simulink model "gm_soc_dvbs2_fpga"  (R2025b)
settings: Solver=FixedStepDiscrete  StartTime=0.0  StopTime=0  RelTol=1e-3
InitFcn:
  | soc_dvbs2_init;
undefined symbols (not defined in the file or in its folder): Add, coefficientsLog, coefficientsSqrt1, coefficientsSqrt2, dataBits, designMultirateFIR, noisePow, Shift, soc_dvbs2_designFIRFilter, soc_dvbs2_txPacketBits, syncWord, txDataOut, txFiltCoeff, XData
libraries: simulink x304, hdlsllib x265, dspsigops x15, dsphdlfiltering2 x8, hdlmdlgenlib x6, dsphdlsigops2 x5, commseqgen3 x5, dsphdlmathfun2 x3, hwlogicconnlib x2, whdledac x2, commhdlcrc x2, whdlutilities x1
(part 1 of 36)
settings Model: DataDictionary=dvbs2hdlReceiverData.sldd  SimulationMode=accelerator  Creator=The MathWorks, Inc.  LastModifiedBy=AEDemo
settings SolverCC: PositivePriorityOrder=on  MaxZcPerStep=1.0
settings DataIOCC: ReturnWorkspaceOutputs=off
settings OptimizationCC: BlockReduction=off  ConditionallyExecuteInputs=off  DefaultParameterBehavior=Inlined  InheritOutputTypeSmallerThanSingle=on  EnhancedBackFolding=on  PassReuseOutputArgsAs=Individual arguments  ZeroExternalMemoryAtStartup=off  ZeroInternalMemoryAtStartup=off  MaxStackSize=64  OptimizeBlockOrder=speed  DifferentSizesBufferReuse=on  OptimizationCustomize=off  EfficientTunableParamExpr=on
settings DebuggingCC: ArtificialAlgebraicLoopMsg=error  InheritedTsInSrcMsg=none  SingleTaskRateTransMsg=error  ParameterTunabilityLossMsg=error  UnconnectedInputMsg=warning  UnconnectedOutputMsg=warning  UnconnectedLineMsg=warning  SubsystemReferenceDiagnosticForUnitTest=warning
settings HardwareCC: ProdBitPerPointer=32.0  ProdBitPerSizeT=32.0  ProdBitPerPtrDiffT=32.0  ProdLargestAtomicFloat=None  ProdIntDivRoundTo=Undefined  ProdEndianess=Unspecified  ProdWordSize=32.0  ProdHWDeviceType=ASIC/FPGA->ASIC/FPGA  TargetBitPerPointer=64.0  TargetBitPerSizeT=64.0  TargetBitPerPtrDiffT=64.0  TargetLongLongMode=on  TargetIntDivRoundTo=Zero  TargetEndianess=LittleEndian  TargetWordSize=64.0  TargetHWDeviceType=Custom Processor->MATLAB Host Computer  ProdEqTarget=off  HardwareBoardFeatureSet=SoCBlockset
settings ModelReferenceCC: EnableRefExpFcnMdlSchedulingChecks=on
settings RTWCC: SystemTargetFile=ert.tlc  HardwareBoard=Xilinx Zynq UltraScale+ RFSoC ZCU111 Evaluation Kit  TLCOptions="-aInlineSetEventsForThisBaseRateFcn=TLC_FALSE -aSuppressMultiTaskScheduler=TLC_FALSE  -aRateBasedStepFcn=0"  TemplateMakefile=ert_default_tmf  Toolchain=Linaro AArch64 Linux v6.3.1  GPUComputeCapability=3.5  DLArmComputeVersion=19.05  Description=Embedded Coder
settings CodeAppCC: ForceParamTrailComments=on  IgnoreCustomStorageClasses=off  OperatorAnnotations=on  SimulinkDataObjDesc=on  SFDataObjDesc=on  InsertBlockDesc=on

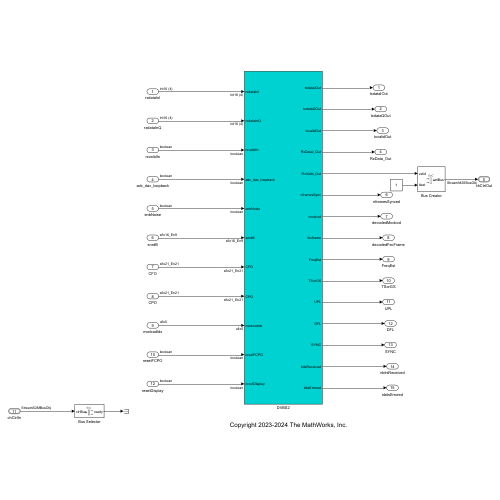
[thumbnail: Simulink's stored preview of the top-level diagram]
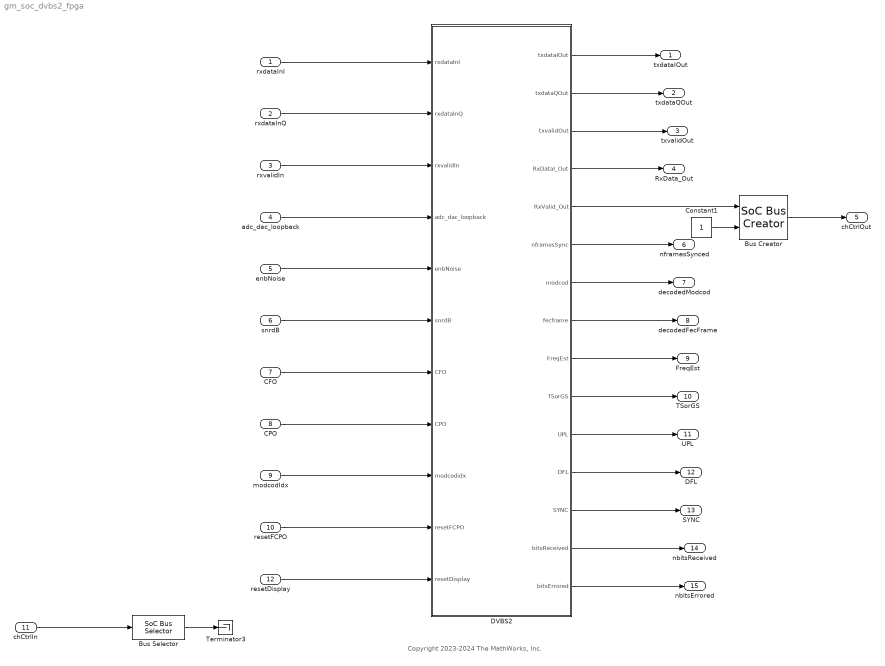
== system gm_soc_dvbs2_fpga ==
  note: Copyright 2023-2024 The MathWorks, Inc.
  rxdataInI : Inport  OutDataTypeStr=int16  PortDimensions=4  LockScale=on
  rxdataInQ : Inport  Port=2  OutDataTypeStr=int16  PortDimensions=4  LockScale=on
  rxvalidIn : Inport  Port=3  OutDataTypeStr=boolean  LockScale=on
  adc_dac_loopback : Inport  Port=4  OutDataTypeStr=boolean  LockScale=on
  enbNoise : Inport  Port=5  OutDataTypeStr=boolean
  snrdB : Inport  Port=6  OutDataTypeStr=fixdt(1,16,9)
  CFO : Inport  Port=7  OutDataTypeStr=fixdt(1,21,21)
  CPO : Inport  Port=8  OutDataTypeStr=fixdt(1,21,21)
  modcodIdx : Inport  Port=9  OutDataTypeStr=fixdt(0,5,0)
  resetFCPO : Inport  Port=10  OutDataTypeStr=boolean
  chCtrlIn : Inport  Port=11  OutDataTypeStr=Bus: StreamS2MBusObj  BusOutputAsStruct=on
  resetDisplay : Inport  Port=12  OutDataTypeStr=boolean
  Bus Creator : hwlogicconnlib/SoC Bus Creator  Protocol=Data stream  ctrltype=Valid
  Bus Selector : hwlogicconnlib/SoC Bus Selector  Protocol=Data stream  ctrltype=Ready
  Constant1 : Constant  OutDataTypeStr=boolean  SampleTime=-1
  DVBS2 : Subsystem
      mask init:
      | coe = reshape(double([0;-4.6183113992051936e-06;-1.117761640887225e-05;-1.8610264502005432e-05;-2.5134586135631012e-05;-2.8494281690666197e-05;-2.6396828793275159e-05;-1.7094212558802163e-05;0;2.3798193576966866e-05;5.1281160242202183e-05;7.7621978262434297e-05;9.6759426664120416e-05;0.00010240229300393402;8.9344614218077133e-05;5.4875700118949183e-05;0;-6.9839082210680138e-05;-0.00014479661323607565;-0.00021158452917708308;-0.00025535069106550544;-0.00026228714374322104;-0.00022258805927027799;-0.00013323230495695704;0;0.00016182578767055206;0.00032846175385096581;0.00047045611576184863;0.00055713851457530922;0.00056212565121518737;0.00046901918553962478;0.00027624866838952986;0;-0.00032564179486838622;-0.00065182310286710399;-0.00092127787309319298;-0.0010772534348943575;-0.0010737727700273478;-0.00088556645390392634;-0.00051581896090765534;0;0.00059548767193795277;0.0011803558710661007;0.0016527320270369871;0.0019152679330965558;0.0018927324805381538;0.0015481870327877928;0.00089470695834941306;0;-0.0010178225878206132;-0.0020037400552054292;-0.0027874356824117317;-0.003210329988021943;-0.0031540624117984395;-0.0025657163651900345;-0.0014750752642111449;0;0.0016624165446378462;0.0032591192839069179;0.004516568581586773;0.0051838984346123896;0.0050774264697459942;0.0041192521414141594;0.00236285754179665;0;-0.0026543507866759182;-0.0051990251084333425;-0.0072020238234656924;-0.0082672928192007358;-0.008103373957295627;-0.006583111539570221;-0.0037839040415292386;0;0.0042781252851152524;0.0084176358598320178;0.011725660574630552;0.013550476647788677;0.013388189369997498;0.010979501242341257;0.006381274941685413;0;-0.007421229604153888;-0.01486456304340213;-0.021143584622178104;-0.02504275058758609;-0.025473530942547201;-0.021627310017882196;-0.013104323383225537;0;0.017065133989980476;0.036978919264451952;0.05823318062093958;0.079072012081405949;0.097675998716952317;0.11236045936950929;0.12176343577287731;0.125;0.12176343577287731;0.11236045936950929;0.097675998716952317;0.079072012081405949;0.05823318062093958;0.036978919264451952;0.017065133989980476;0;-0.013104323383225537;-0.021627310017882196;-0.025473530942547201;-0.02504275058758609;-0.021143584622178104;-0.01486456304340213;-0.007421229604153888;0;0.006381274941685413;0.010979501242341257;0.013388189369997498;0.013550476647788677;0.011725660574630552;0.0084176358598320178;0.0042781252851152524;0;-0.0037839040415292386;-0.006583111539570221;-0.008103373957295627;-0.0082672928192007358;-0.0072020238234656924;-0.0051990251084333425;-0.0026543507866759182;0;0.00236285754179665;0.0041192521414141594;0.0050774264697459942;0.0051838984346123896;0.004516568581586773;0.0032591192839069179;0.0016624165446378462;0;-0.0014750752642111449;-0.0025657163651900345;-0.0031540624117984395;-0.003210329988021943;-0.0027874356824117317;-0.0020037400552054292;-0.0010178225878206132;0;0.00089470695834941306;0.0015481870327877928;0.0018927324805381538;0.0019152679330965558;0.0016527320270369871;0.0011803558710661007;0.00059548767193795277;0;-0.00051581896090765534;-0.00088556645390392634;-0.0010737727700273478;-0.0010772534348943575;-0.00092127787309319298;-0.00065182310286710399;-0.00032564179486838622;0;0.00027624866838952986;0.00046901918553962478;0.00056212565121518737;0.00055713851457530922;0.00047045611576184863;0.00032846175385096581;0.00016182578767055206;0;-0.00013323230495695704;-0.00022258805927027799;-0.00026228714374322104;-0.00025535069106550544;-0.00021158452917708308;-0.00014479661323607565;-6.9839082210680138e-05;0;5.4875700118949183e-05;8.9344614218077133e-05;0.00010240229300393402;9.6759426664120416e-05;7.7621978262434297e-05;5.1281160242202183e-05;2.3798193576966866e-05;0;-1.7094212558802163e-05;-2.6396828793275159e-05;-2.8494281690666197e-05;-2.5134586135631012e-05;-1.8610264502005432e-05;-1.117761640887225e-05;-4.6183113992051936e-06]), [1  192]);
      | interp_coeff = reshape(double([0;-2.5762581491757149e-05;-5.8831821680514759e-05;-9.3312161185059878e-05;-0.00012086163085409433;-0.00013205270976779482;-0.00011834743116057382;-7.4366825754989437e-05;0;9.8160915307191784e-05;0.00020653032645552219;0.00030569884691874328;0.00037312606030348193;0.00038710567399410266;0.00033143343994865174;0.00019995023815725909;0;-0.00024611644953130535;-0.00050237406876756942;-0.00072320914773199184;-0.00086038268936497941;-0.00087166788797456607;-0.00073000105198961778;-0.00043141174353976327;0;0.00051149159396842369;0.0010263594832950844;0.0014538625812232689;0.0017033853517477954;0.0017008871462745852;0.0014049583413437243;0.00081947197501865956;0;-0.00094810607847870226;-0.0018808492888220838;-0.0026352624613329868;-0.0030553081816828832;-0.0030202428411423995;-0.0024707286522091098;-0.0014277474612946694;0;0.0016230413454147042;0.0031930796109812462;0.0044380259174111297;0.0051056581078908472;0.0050093785155702775;0.0040683784677133959;0.0023345651421505286;0;-0.0026187539064786284;-0.0051193984472911441;-0.0070718134335119327;-0.0080873994108355395;-0.0078893031903380026;-0.0063716582505391091;-0.0036365506713397764;0;0.0040374115839547997;0.0078540829737719763;0.010798012443441477;0.012292073245047443;0.011937778189025024;0.0095999760380976757;0.0054563636732276643;0;-0.0060102816730613498;-0.011648449375858055;-0.015957241826634484;-0.018102591848754991;-0.017522692405904365;-0.014046537497763033;-0.007959475987989087;0;0.008718104923122711;0.01685235137753412;0.023029139138304663;0.026064622673058715;0.025174843574555367;0.020139852028642682;0.011390947438140097;0;-0.012436079757686049;-0.024006222786136334;-0.032765654100451284;-0.03704666586468406;-0.035752212682362922;-0.028583560689952235;-0.01615969653056519;0;0.017638825193237648;0.034058051458235795;0.046508756928501517;0.052626172604575812;0.050841305470613003;0.040702766275549772;0.023050307008179838;0;-0.025272869236065459;-0.048936761752801212;-0.067046073615192756;-0.07615058129553684;-0.073883911648887329;-0.05943876854292833;-0.033846317708509245;0;0.037602423644390599;0.073384893960547079;0.10143269424548541;0.11635564505557951;0.11415986456169339;0.093003185804921784;0.053716748922668422;0;-0.061764245016254132;-0.12307869991479406;-0.17423577931097833;-0.20545948334743191;-0.20814945771861357;-0.17607037667070338;-0.10632880802090262;0;0.13769341192513965;0.29769467708537439;0.46790031420225453;0.63434243500199439;0.78263423378671237;0.89951021019816191;0.97427716367867034;1;0.97427716367867034;0.89951021019816191;0.78263423378671237;0.63434243500199439;0.46790031420225453;0.29769467708537439;0.13769341192513965;0;-0.10632880802090262;-0.17607037667070338;-0.20814945771861357;-0.20545948334743191;-0.17423577931097833;-0.12307869991479406;-0.061764245016254132;0;0.053716748922668422;0.093003185804921784;0.11415986456169339;0.11635564505557951;0.10143269424548541;0.073384893960547079;0.037602423644390599;0;-0.033846317708509245;-0.05943876854292833;-0.073883911648887329;-0.07615058129553684;-0.067046073615192756;-0.048936761752801212;-0.025272869236065459;0;0.023050307008179838;0.040702766275549772;0.050841305470613003;0.052626172604575812;0.046508756928501517;0.034058051458235795;0.017638825193237648;0;-0.01615969653056519;-0.028583560689952235;-0.035752212682362922;-0.03704666586468406;-0.032765654100451284;-0.024006222786136334;-0.012436079757686049;0;0.011390947438140097;0.020139852028642682;0.025174843574555367;0.026064622673058715;0.023029139138304663;0.01685235137753412;0.008718104923122711;0;-0.007959475987989087;-0.014046537497763033;-0.017522692405904365;-0.018102591848754991;-0.015957241826634484;-0.011648449375858055;-0.0060102816730613498;0;0.0054563636732276643;0.0095999760380976757;0.011937778189025024;0.012292073245047443;0.010798012443441477;0.0078540829737719763;0.0040374115839547997;0;-0.0036365506713397764;-0.0063716582505391091;-0.0078893031903380026;-0.0080873994108355395;-0.0070718134335119327;-0.0051193984472911441;-0.0026187539064786284;0;0.0023345651421505286;0.0040683784677133959;0.0050093785155702775;0.0051056581078908472;0.0044380259174111297;0.0031930796109812462;0.0016230413454147042;0;-0.0014277474612946694;-0.0024707286522091098;-0.0030202428411423995;-0.0030553081816828832;-0.0026352624613329868;-0.0018808492888220838;-0.00094810607847870226;0;0.00081947197501865956;0.0014049583413437243;0.0017008871462745852;0.0017033853517477954;0.0014538625812232689;0.0010263594832950844;0.00051149159396842369;0;-0.00043141174353976327;-0.00073000105198961778;-0.00087166788797456607;-0.00086038268936497941;-0.00072320914773199184;-0.00050237406876756942;-0.00024611644953130535;0;0.00019995023815725909;0.00033143343994865174;0.00038710567399410266;0.00037312606030348193;0.00030569884691874328;0.00020653032645552219;9.8160915307191784e-05;0;-7.4366825754989437e-05;-0.00011834743116057382;-0.00013205270976779482;-0.00012086163085409433;-9.3312161185059878e-05;-5.8831821680514759e-05;-2.5762581491757149e-05]), [1  256]);
  Terminator3 : Terminator
  txdataIOut : Outport
  txdataQOut : Outport  Port=2
  txvalidOut : Outport  Port=3
  RxData_Out : Outport  Port=4
  chCtrlOut : Outport  Port=5  OutDataTypeStr=Bus: StreamM2SBusObj  VectorParamsAs1DForOutWhenUnconnected=off  BusOutputAsStruct=on
  nframesSynced : Outport  Port=6
  decodedModcod : Outport  Port=7
  decodedFecFrame : Outport  Port=8
  FreqEst : Outport  Port=9
  TSorGS : Outport  Port=10
  UPL : Outport  Port=11
  DFL : Outport  Port=12
  SYNC : Outport  Port=13
  nbitsReceived : Outport  Port=14
  nbitsErrored : Outport  Port=15
  wires:
  resetDisplay/1 -> DVBS2/11(resetDisplay)
  DVBS2/15(bitsErrored) -> nbitsErrored/1
  DVBS2/14(bitsReceived) -> nbitsReceived/1
  DVBS2/12(DFL) -> DFL/1
  DVBS2/10(TSorGS) -> TSorGS/1
  DVBS2/13(SYNC) -> SYNC/1
  DVBS2/11(UPL) -> UPL/1
  DVBS2/2(txdataQOut) -> txdataQOut/1
  DVBS2/1(txdataIOut) -> txdataIOut/1
  CFO/1 -> DVBS2/7(CFO)
  Bus Selector/1 -> Terminator3/1
  chCtrlIn/1 -> Bus Selector/1
  Constant1/1 -> Bus Creator/2
  DVBS2/5(RxValid_Out) -> Bus Creator/1
  Bus Creator/1 -> chCtrlOut/1
  DVBS2/4(RxDataI_Out) -> RxData_Out/1
  resetFCPO/1 -> DVBS2/10(resetFCPO)
  DVBS2/9(FreqEst) -> FreqEst/1
  DVBS2/8(fecframe) -> decodedFecFrame/1
  DVBS2/7(modcod) -> decodedModcod/1
  DVBS2/6(nframesSync) -> nframesSynced/1
  DVBS2/3(txvalidOut) -> txvalidOut/1
  enbNoise/1 -> DVBS2/5(enbNoise)
  modcodIdx/1 -> DVBS2/9(modcodidx)
  CPO/1 -> DVBS2/8(CPO)
  snrdB/1 -> DVBS2/6(snrdB)
  adc_dac_loopback/1 -> DVBS2/4(adc_dac_loopback)
  rxvalidIn/1 -> DVBS2/3(rxvalidIn)
  rxdataInQ/1 -> DVBS2/2(rxdataInQ)
  rxdataInI/1 -> DVBS2/1(rxdataInI)

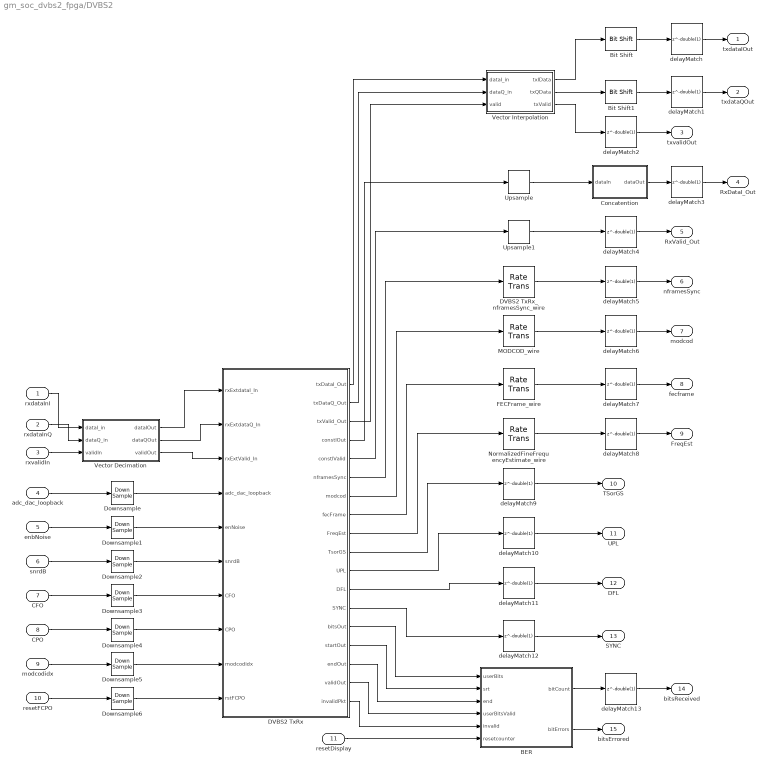
== system gm_soc_dvbs2_fpga/DVBS2 ==
  rxdataInI : Inport  OutDataTypeStr=int16  PortDimensions=[4]  SampleTime=7.8125e-09
  rxdataInQ : Inport  Port=2  OutDataTypeStr=int16  PortDimensions=[4]  SampleTime=7.8125e-09
  rxvalidIn : Inport  Port=3  OutDataTypeStr=boolean  PortDimensions=1  SampleTime=7.8125e-09
  adc_dac_loopback : Inport  Port=4  OutDataTypeStr=boolean  PortDimensions=1  SampleTime=7.8125e-09
  enbNoise : Inport  Port=5  OutDataTypeStr=boolean  PortDimensions=1  SampleTime=7.8125e-09
  snrdB : Inport  Port=6  OutDataTypeStr=fixdt(1, 16, 9)  PortDimensions=1  SampleTime=7.8125e-09
  CFO : Inport  Port=7  OutDataTypeStr=fixdt(1, 21, 21)  PortDimensions=1  SampleTime=7.8125e-09
  CPO : Inport  Port=8  OutDataTypeStr=fixdt(1, 21, 21)  PortDimensions=1  SampleTime=7.8125e-09
  modcodidx : Inport  Port=9  OutDataTypeStr=fixdt(0, 5, 0)  PortDimensions=1  SampleTime=7.8125e-09
  resetFCPO : Inport  Port=10  OutDataTypeStr=boolean  PortDimensions=1  SampleTime=7.8125e-09
  resetDisplay : Inport  Port=11  OutDataTypeStr=boolean  PortDimensions=1  SampleTime=7.8125e-09
  BER : Subsystem
  Bit Shift : hdlsllib/Logic and Bit Operations/Bit Shift  mode=Shift Left Logical  N=double(2)
  Bit Shift1 : hdlsllib/Logic and Bit Operations/Bit Shift  mode=Shift Left Logical  N=double(2)
  Concatention : Subsystem
  DVBS2 TxRx : Subsystem
  DVBS2 TxRx_nframesSync_wire : RateTransition  Integrity=off  Deterministic=off  OutPortSampleTimeOpt=Multiple of input port sample time  OutPortSampleTimeMultiple=1/32
  Downsample{,1..6} (7 alike) : DownSample  N=double(8)  phase=double(0)  RateOptions=Allow multirate processing  AllowArbitraryFixedInput=on
  FECFrame_wire : RateTransition  Integrity=off  Deterministic=off  OutPortSampleTimeOpt=Multiple of input port sample time  OutPortSampleTimeMultiple=1/32
  MODCOD_wire : RateTransition  Integrity=off  Deterministic=off  OutPortSampleTimeOpt=Multiple of input port sample time  OutPortSampleTimeMultiple=1/32
  NormalizedFineFrequencyEstimate_wire : RateTransition  Integrity=off  Deterministic=off  OutPortSampleTimeOpt=Multiple of input port sample time  OutPortSampleTimeMultiple=1/32
  Upsample : dspsigops/Upsample  FactorSource=Dialog parameter  N=double(32)  Nmax=16  phase=double(0)  RateOptions=Allow multirate processing  ic=0  mode=Unused parameter value
  Upsample1 : dspsigops/Upsample  FactorSource=Dialog parameter  N=double(32)  Nmax=16  phase=double(0)  RateOptions=Allow multirate processing  ic=0  mode=Unused parameter value
  Vector Decimation : Subsystem
  Vector Interpolation : Subsystem
  delayMatch{,1..13} (14 alike) : Delay  DelayLength=double(1)  InitialCondition=0  SampleTime=7.8125e-09
  txdataIOut : Outport  SampleTime=7.8125e-09
  txdataQOut : Outport  Port=2  SampleTime=7.8125e-09
  txvalidOut : Outport  Port=3  SampleTime=7.8125e-09
  RxDataI_Out : Outport  Port=4  SampleTime=7.8125e-09
  RxValid_Out : Outport  Port=5  SampleTime=7.8125e-09
  nframesSync : Outport  Port=6  SampleTime=7.8125e-09
  modcod : Outport  Port=7  SampleTime=7.8125e-09
  fecframe : Outport  Port=8  SampleTime=7.8125e-09
  FreqEst : Outport  Port=9  SampleTime=7.8125e-09
  TSorGS : Outport  Port=10  SampleTime=7.8125e-09
  UPL : Outport  Port=11  SampleTime=7.8125e-09
  DFL : Outport  Port=12  SampleTime=7.8125e-09
  SYNC : Outport  Port=13  SampleTime=7.8125e-09
  bitsReceived : Outport  Port=14  SampleTime=7.8125e-09
  bitsErrored : Outport  Port=15  SampleTime=7.8125e-09
  wires:
  Downsample5/1 -> DVBS2 TxRx/9(modcodidx)
  enbNoise/1 -> Downsample1/1
  DVBS2 TxRx_nframesSync_wire/1 -> delayMatch5/1
  rxdataInI/1 -> Vector Decimation/1(dataI_in)
  DVBS2 TxRx/7(modcod) -> MODCOD_wire/1
  CPO/1 -> Downsample4/1
  CFO/1 -> Downsample3/1
  DVBS2 TxRx/2(txDataQ_Out) -> Vector Interpolation/2(dataQ_in)
  Upsample1/1 -> delayMatch4/1
  DVBS2 TxRx/5(constlValid) -> Upsample1/1
  snrdB/1 -> Downsample2/1
  DVBS2 TxRx/3(txValid_Out) -> Vector Interpolation/3(valid)
  adc_dac_loopback/1 -> Downsample/1
  NormalizedFineFrequencyEstimate_wire/1 -> delayMatch8/1
  resetDisplay/1 -> BER/6(resetcounter)
  DVBS2 TxRx/6(nframesSync) -> DVBS2 TxRx_nframesSync_wire/1
  rxvalidIn/1 -> Vector Decimation/3(validIn)
  Bit Shift1/1 -> delayMatch1/1
  DVBS2 TxRx/1(txDataI_Out) -> Vector Interpolation/1(dataI_in)
  resetFCPO/1 -> Downsample6/1
  rxdataInQ/1 -> Vector Decimation/2(dataQ_in)
  DVBS2 TxRx/4(constlOut) -> Upsample/1
  modcodidx/1 -> Downsample5/1
  Vector Decimation/1(dataIOut) -> DVBS2 TxRx/1(rxExtdataI_In)
  Vector Decimation/2(dataQOut) -> DVBS2 TxRx/2(rxExtdataQ_In)
  MODCOD_wire/1 -> delayMatch6/1
  Vector Decimation/3(validOut) -> DVBS2 TxRx/3(rxExtValid_In)
  FECFrame_wire/1 -> delayMatch7/1
  Downsample/1 -> DVBS2 TxRx/4(adc_dac_loopback)
  Downsample1/1 -> DVBS2 TxRx/5(enNoise)
  Downsample2/1 -> DVBS2 TxRx/6(snrdB)
  Downsample4/1 -> DVBS2 TxRx/8(CPO)
  Downsample3/1 -> DVBS2 TxRx/7(CFO)
  Downsample6/1 -> DVBS2 TxRx/10(rstFCPO)
  DVBS2 TxRx/8(fecFrame) -> FECFrame_wire/1
  delayMatch11/1 -> DFL/1
  DVBS2 TxRx/17(validOut) -> BER/4(userBitsValid)
  DVBS2 TxRx/9(FreqEst) -> NormalizedFineFrequencyEstimate_wire/1
  DVBS2 TxRx/10(TsorGS) -> delayMatch9/1
  delayMatch9/1 -> TSorGS/1
  DVBS2 TxRx/18(invalidPkt) -> BER/5(invalid)
  delayMatch7/1 -> fecframe/1
  DVBS2 TxRx/11(UPL) -> delayMatch10/1
  delayMatch5/1 -> nframesSync/1
  DVBS2 TxRx/12(DFL) -> delayMatch11/1
  DVBS2 TxRx/13(SYNC) -> delayMatch12/1
  DVBS2 TxRx/14(bitsOut) -> BER/1(userBits)
  DVBS2 TxRx/15(startOut) -> BER/2(srt)
  Vector Interpolation/2(txQData) -> Bit Shift1/1
  delayMatch13/1 -> bitsReceived/1
  DVBS2 TxRx/16(endOut) -> BER/3(end)
  delayMatch6/1 -> modcod/1
  Vector Interpolation/1(txIData) -> Bit Shift/1
  Vector Interpolation/3(txValid) -> delayMatch2/1
  Upsample/1 -> Concatention/1(dataIn)
  delayMatch10/1 -> UPL/1
  delayMatch12/1 -> SYNC/1
  BER/1(bitCount) -> delayMatch13/1
  BER/2(bitErrors) -> bitsErrored/1
  Bit Shift/1 -> delayMatch/1
  delayMatch2/1 -> txvalidOut/1
  Concatention/1(dataOut) -> delayMatch3/1
  delayMatch4/1 -> RxValid_Out/1
  delayMatch8/1 -> FreqEst/1
  delayMatch/1 -> txdataIOut/1
  delayMatch1/1 -> txdataQOut/1
  delayMatch3/1 -> RxDataI_Out/1

== system gm_soc_dvbs2_fpga/DVBS2/BER ==
  userBits : Inport  OutDataTypeStr=boolean  PortDimensions=1  SampleTime=7.8125e-09
  srt : Inport  Port=2  OutDataTypeStr=boolean  PortDimensions=1  SampleTime=7.8125e-09
  end : Inport  Port=3  OutDataTypeStr=boolean  PortDimensions=1  SampleTime=7.8125e-09
  userBitsValid : Inport  Port=4  OutDataTypeStr=boolean  PortDimensions=1  SampleTime=7.8125e-09
  invalid : Inport  Port=5  OutDataTypeStr=boolean  PortDimensions=1  SampleTime=7.8125e-09
  resetcounter : Inport  Port=6  OutDataTypeStr=boolean  PortDimensions=1  SampleTime=7.8125e-09
  Compare To Constant : simulink/Logic and Bit Operations/Compare To Constant  relop===  const="fi(0,0,32,0,\"hex\",\"00000000\")"  OutDataTypeStr=boolean
  Data Type Conversion1 : DataTypeConversion  OutDataTypeStr=boolean  SampleTime=7.8125e-09  SaturateOnIntegerOverflow=off  RndMeth=Floor
  Delay : Delay  DelayLength=double(1)  InitialCondition=0  SampleTime=7.8125e-09
  Delay1 : Delay  DelayLength=double(1)  InitialCondition=0  SampleTime=7.8125e-09
  Delay4 : Delay  DelayLength=double(1550)  InitialCondition=0  SampleTime=7.8125e-09
  Delay5 : Delay  DelayLength=double(1550)  InitialCondition=0  SampleTime=7.8125e-09
  Delay6 : Delay  DelayLength=double(1550)  InitialCondition=0  SampleTime=7.8125e-09
  HDL Counter : hdlsllib/Sources/HDL Counter  CountType=Free running  CountInit=0  CountStep=1  CountMax=25  CountFromType=Initial value  CountFrom=0  CountResetPort=on  CountLoadPort=off  CountEnbPort=on  CountDirPort=off  CountHitOutputPort=off  CountDataType=Unsigned  CountWordLen=32  CountFracLen=0  CountSampTime=1
  HDL Counter1 : hdlsllib/Sources/HDL Counter  CountType=Free running  CountInit=0  CountStep=1  CountMax=25  CountFromType=Initial value  CountFrom=0  CountResetPort=on  CountLoadPort=off  CountEnbPort=on  CountDirPort=off  CountHitOutputPort=off  CountDataType=Unsigned  CountWordLen=32  CountFracLen=0  CountSampTime=1
  Logical Operator : Logic  AllPortsSameDT=off  OutDataTypeStr=boolean  SampleTime=7.8125e-09
  Logical Operator1 : Logic  Operator=OR  AllPortsSameDT=off  OutDataTypeStr=boolean  SampleTime=7.8125e-09
  Logical Operator2 : Logic  Operator=NOT  Inputs=1  AllPortsSameDT=off  OutDataTypeStr=boolean  SampleTime=7.8125e-09
  Logical Operator3 : Logic  AllPortsSameDT=off  OutDataTypeStr=boolean  SampleTime=7.8125e-09
  Relational Operator : RelationalOperator  Operator=~=  OutDataTypeStr=boolean  SampleTime=7.8125e-09  InputSameDT=off
  Send Payload Data : Subsystem
  Unit Delay Enabled Synchronous : hdlsllib/Discrete/Unit Delay Enabled Synchronous  InitialCondition=double(0)  SampleTime=-1
  Unit Delay Enabled Synchronous1 : hdlsllib/Discrete/Unit Delay Enabled Synchronous  InitialCondition=double(0)  SampleTime=-1
  delayMatch : Delay  DelayLength=double(1)  InitialCondition=0  SampleTime=7.8125e-09
  delayMatch1 : Delay  DelayLength=double(1)  InitialCondition=0  SampleTime=7.8125e-09
  delayMatch2 : Delay  DelayLength=double(1)  InitialCondition=0  SampleTime=7.8125e-09
  bitCount : Outport  SampleTime=7.8125e-09  VectorParamsAs1DForOutWhenUnconnected=off
  bitErrors : Outport  Port=2  SampleTime=7.8125e-09  VectorParamsAs1DForOutWhenUnconnected=off
  wires:
  userBitsValid/1 -> Delay4/1
  Data Type Conversion1/1 -> Relational Operator/2
  invalid/1 -> Unit Delay Enabled Synchronous/1
  srt/1 -> Delay6/1
  end/1 -> Unit Delay Enabled Synchronous/2
  Unit Delay Enabled Synchronous/1 -> Logical Operator2/1
  Logical Operator/1 -> HDL Counter/2
  delayMatch2/1 -> HDL Counter/1
  Logical Operator2/1 -> Unit Delay Enabled Synchronous1/1
  Delay4/1 -> Delay1/1
  Delay6/1 -> Send Payload Data/1(rst), Unit Delay Enabled Synchronous1/2
  Unit Delay Enabled Synchronous1/1 -> Logical Operator3/1
  Delay1/1 -> Logical Operator3/2
  userBits/1 -> Delay5/1
  resetcounter/1 -> Logical Operator1/2, HDL Counter1/1
  Logical Operator3/1 -> delayMatch1/1, HDL Counter1/2, Send Payload Data/2(nxtBit)
  Delay5/1 -> Delay/1
  HDL Counter1/1 -> Compare To Constant/1, bitCount/1
  Delay/1 -> delayMatch/1
  Send Payload Data/1(dataIn) -> Data Type Conversion1/1
  Compare To Constant/1 -> Logical Operator1/1
  delayMatch/1 -> Relational Operator/1
  Logical Operator1/1 -> delayMatch2/1
  delayMatch1/1 -> Logical Operator/1
  Relational Operator/1 -> Logical Operator/2
  HDL Counter/1 -> bitErrors/1

== system gm_soc_dvbs2_fpga/DVBS2/Concatention ==
  dataIn : Inport  OutDataTypeStr=fixdt(1, 18, 14)  PortDimensions=1  SampleTime=7.8125e-09
      settings: SignalType=complex
  Bit Concat : hdlsllib/Logic and Bit Operations/Bit Concat  numInputs=2
  Complex to Real-Imag1 : ComplexToRealImag
  Data Type Conversion : DataTypeConversion  OutDataTypeStr=fixdt(1,16,12)  SaturateOnIntegerOverflow=off  RndMeth=Floor
  Data Type Conversion1 : DataTypeConversion  OutDataTypeStr=int16  ConvertRealWorld=Stored Integer (SI)  SaturateOnIntegerOverflow=off  RndMeth=Floor
  dataOut : Outport  SampleTime=7.8125e-09
  wires:
  dataIn/1 -> Data Type Conversion/1
  Bit Concat/1 -> dataOut/1
  Complex to Real-Imag1/2 -> Bit Concat/2
  Complex to Real-Imag1/1 -> Bit Concat/1
  Data Type Conversion1/1 -> Complex to Real-Imag1/1
  Data Type Conversion/1 -> Data Type Conversion1/1

== system gm_soc_dvbs2_fpga/DVBS2/DVBS2 TxRx ==
  rxExtdataI_In : Inport  OutDataTypeStr=int16  PortDimensions=1  SampleTime=7.8125e-09
  rxExtdataQ_In : Inport  Port=2  OutDataTypeStr=int16  PortDimensions=1  SampleTime=7.8125e-09
  rxExtValid_In : Inport  Port=3  OutDataTypeStr=boolean  PortDimensions=1  SampleTime=7.8125e-09
  adc_dac_loopback : Inport  Port=4  OutDataTypeStr=boolean  PortDimensions=1  SampleTime=6.25e-08
  enNoise : Inport  Port=5  OutDataTypeStr=boolean  PortDimensions=1  SampleTime=6.25e-08
  snrdB : Inport  Port=6  OutDataTypeStr=fixdt(1, 16, 9)  PortDimensions=1  SampleTime=6.25e-08
  CFO : Inport  Port=7  OutDataTypeStr=fixdt(1, 21, 21)  PortDimensions=1  SampleTime=6.25e-08
  CPO : Inport  Port=8  OutDataTypeStr=fixdt(1, 21, 21)  PortDimensions=1  SampleTime=6.25e-08
  modcodidx : Inport  Port=9  OutDataTypeStr=fixdt(0, 5, 0)  PortDimensions=1  SampleTime=6.25e-08
  rstFCPO : Inport  Port=10  OutDataTypeStr=boolean  PortDimensions=1  SampleTime=6.25e-08
  Bus Selector : BusSelector  OutputSignals=TSorGS,UPL,DFL,SYNC
  Channel : Subsystem
  Complex to Real-Imag : ComplexToRealImag
  DVB-S2 HDL Receiver : Subsystem
  Digital Automatic Gain Control : Subsystem  mask{desiredOutputPower=double(0.25), stepSize=double(0.0005)}
      mask prompts: desiredOutputPower "Desired output power:"; stepSize "Adaptation step size:"
      mask init:
      | desiredOutputPower = double(0.25);
      | slopeAdj = double(1);
      | stepSize = double(0.0005);
      mask Display:
      | dispstr1 = 'Digital AGC';
      | disp(dispstr1);
  Downsample7 : DownSample  N=4  RateOptions=Allow multirate processing
  LUT Based Tx : Subsystem
  Prepare Inputs : Subsystem
  Prepare Outputs : Subsystem
  Real-Imag to Complex : RealImagToComplex
  Switch : Switch  Criteria=u2 ~= 0  OutDataTypeStr=fixdt(1, 18, 15)  SaturateOnIntegerOverflow=off  InputSameDT=off
  Switch1 : Switch  Criteria=u2 ~= 0  OutDataTypeStr=boolean  SaturateOnIntegerOverflow=off  InputSameDT=off
  txDataI_Out : Outport  SampleTime=7.8125e-09
  txDataQ_Out : Outport  Port=2  SampleTime=7.8125e-09
  txValid_Out : Outport  Port=3  SampleTime=7.8125e-09
  constlOut : Outport  Port=4  SampleTime=2.5e-07
  constlValid : Outport  Port=5  SampleTime=2.5e-07
  nframesSync : Outport  Port=6  SampleTime=2.5e-07
  modcod : Outport  Port=7  SampleTime=2.5e-07
  fecFrame : Outport  Port=8  SampleTime=2.5e-07
  FreqEst : Outport  Port=9  SampleTime=2.5e-07
  TsorGS : Outport  Port=10  SampleTime=7.8125e-09
  UPL : Outport  Port=11  SampleTime=7.8125e-09
  DFL : Outport  Port=12  SampleTime=7.8125e-09
  SYNC : Outport  Port=13  SampleTime=7.8125e-09
  bitsOut : Outport  Port=14  SampleTime=7.8125e-09
  startOut : Outport  Port=15  SampleTime=7.8125e-09
  endOut : Outport  Port=16  SampleTime=7.8125e-09
  validOut : Outport  Port=17  SampleTime=7.8125e-09
  invalidPkt : Outport  Port=18  SampleTime=7.8125e-09
  wires:
  rxExtdataQ_In/1 -> Real-Imag to Complex/2
  rstFCPO/1 -> DVB-S2 HDL Receiver/3(rstFCPO)
  rxExtdataI_In/1 -> Real-Imag to Complex/1
  modcodidx/1 -> Downsample7/1
  Downsample7/1 -> LUT Based Tx/1(modcodidx)
  Real-Imag to Complex/1 -> Prepare Inputs/1(rxData)
  LUT Based Tx/1(txDataOut) -> Channel/1(txDataOut), Prepare Outputs/1(txData)
  DVB-S2 HDL Receiver/2(syncSymbValid) -> constlValid/1
  LUT Based Tx/2(txValidOut) -> Channel/2(txValidOut), Prepare Outputs/2(txvalid)
  DVB-S2 HDL Receiver/9(endOut) -> endOut/1
  Switch/1 -> Digital Automatic Gain Control/1(dataIn)
  rxExtValid_In/1 -> Prepare Inputs/2(rxValid)
  DVB-S2 HDL Receiver/8(startOut) -> startOut/1
  snrdB/1 -> Channel/3(snrdB)
  DVB-S2 HDL Receiver/7(bitsOut) -> bitsOut/1
  enNoise/1 -> Channel/4(enNoise)
  DVB-S2 HDL Receiver/5(fecFrame) -> fecFrame/1
  CFO/1 -> Channel/5(CFO)
  DVB-S2 HDL Receiver/6(fineFreqEst) -> FreqEst/1
  CPO/1 -> Channel/6(CPO)
  Prepare Outputs/1(txDataOut) -> Complex to Real-Imag/1
  Prepare Outputs/2(txValidOut) -> txValid_Out/1
  Prepare Inputs/1(rxDataOut) -> Switch/1
  Prepare Inputs/2(rxValidOut) -> Switch1/1
  DVB-S2 HDL Receiver/10(validOut) -> validOut/1
  adc_dac_loopback/1 -> Switch1/2, Switch/2
  Channel/1(dataOut) -> Switch/3
  Bus Selector/3 -> DFL/1
  Channel/2(validOut) -> Switch1/3
  Complex to Real-Imag/1 -> txDataI_Out/1
  Complex to Real-Imag/2 -> txDataQ_Out/1
  Switch1/1 -> Digital Automatic Gain Control/2(validIn)
  Digital Automatic Gain Control/1(dataOut) -> DVB-S2 HDL Receiver/1(dataIn)
  Bus Selector/4 -> SYNC/1
  Digital Automatic Gain Control/2(validOut) -> DVB-S2 HDL Receiver/2(validIn)
  DVB-S2 HDL Receiver/1(syncSymb) -> constlOut/1
  DVB-S2 HDL Receiver/11(invalidPkt) -> invalidPkt/1
  DVB-S2 HDL Receiver/3(numSynced) -> nframesSync/1
  DVB-S2 HDL Receiver/12(BBheaderParams) -> Bus Selector/1
  DVB-S2 HDL Receiver/4(MODCOD) -> modcod/1
  Bus Selector/1 -> TsorGS/1
  Bus Selector/2 -> UPL/1

== system gm_soc_dvbs2_fpga/DVBS2/Vector Decimation ==
  dataI_in : Inport  OutDataTypeStr=int16  PortDimensions=[4]  SampleTime=7.8125e-09
  dataQ_in : Inport  Port=2  OutDataTypeStr=int16  PortDimensions=[4]  SampleTime=7.8125e-09
  validIn : Inport  Port=3  OutDataTypeStr=boolean  PortDimensions=1  SampleTime=7.8125e-09
  Bit Shift : hdlsllib/Logic and Bit Operations/Bit Shift  mode=Shift Left Logical  N=4
  Complex to Real-Imag : ComplexToRealImag
  Vector Decimation : Subsystem
  dataIOut : Outport  SampleTime=7.8125e-09
  dataQOut : Outport  Port=2  SampleTime=7.8125e-09
  validOut : Outport  Port=3  SampleTime=7.8125e-09
  wires:
  Vector Decimation/2(vout) -> validOut/1
  validIn/1 -> Vector Decimation/3(vin)
  dataI_in/1 -> Vector Decimation/1(din_real)
  Vector Decimation/1(dout) -> Bit Shift/1
  dataQ_in/1 -> Vector Decimation/2(din_img)
  Complex to Real-Imag/2 -> dataQOut/1
  Bit Shift/1 -> Complex to Real-Imag/1
  Complex to Real-Imag/1 -> dataIOut/1

== system gm_soc_dvbs2_fpga/DVBS2/Vector Interpolation ==
  dataI_in : Inport  OutDataTypeStr=int16  PortDimensions=1  SampleTime=7.8125e-09
  dataQ_in : Inport  Port=2  OutDataTypeStr=int16  PortDimensions=1  SampleTime=7.8125e-09
  valid : Inport  Port=3  OutDataTypeStr=boolean  PortDimensions=1  SampleTime=7.8125e-09
  Complex to Real-Imag : ComplexToRealImag
  Data Type Conversion3 : DataTypeConversion  OutDataTypeStr=int16  SaturateOnIntegerOverflow=off  RndMeth=Floor
  Data Type Conversion4 : DataTypeConversion  OutDataTypeStr=int16  SaturateOnIntegerOverflow=off  RndMeth=Floor
  Extract Bits1 : simulink/Logic and Bit Operations/Extract Bits  bitsToExtract=Range starting with most significant bit  numBits=12  bitIdxRange=[0 7]  outScalingMode=Treat bit field as an integer
  Extract Bits2 : simulink/Logic and Bit Operations/Extract Bits  bitsToExtract=Range starting with most significant bit  numBits=12  bitIdxRange=[0 7]  outScalingMode=Treat bit field as an integer
  FIR Interpolator : dsphdlfiltering2/FIR Interpolator  NumeratorSource=Property  Numerator=designMultirateFIR(4,1,16)  NumeratorPrototype=[]  FilterStructure=Direct form systolic  InterpolationFactor=4  NumCycles=1  OptimizeSymmCoeff=off  SimulateUsing=Code generation  roundingMode=Floor  overflowMode=off  CoefficientsDataTypeStr=Inherit: Same word length as input  OutputDataTypeStr=fixdt(1,16,0)  ResetInputPort=off  HDLGlobalReset=off
  FIR Interpolator_term2 : Terminator
  Real-Imag to Complex : RealImagToComplex
  txIData : Outport  SampleTime=7.8125e-09
  txQData : Outport  Port=2  SampleTime=7.8125e-09
  txValid : Outport  Port=3  SampleTime=7.8125e-09
  wires:
  FIR Interpolator/3 -> FIR Interpolator_term2/1
  valid/1 -> FIR Interpolator/2
  dataI_in/1 -> Extract Bits1/1
  dataQ_in/1 -> Extract Bits2/1
  Data Type Conversion3/1 -> Real-Imag to Complex/1
  Extract Bits2/1 -> Data Type Conversion4/1
  Extract Bits1/1 -> Data Type Conversion3/1
  Data Type Conversion4/1 -> Real-Imag to Complex/2
  Real-Imag to Complex/1 -> FIR Interpolator/1
  FIR Interpolator/1 -> Complex to Real-Imag/1
  FIR Interpolator/2 -> txValid/1
  Complex to Real-Imag/1 -> txIData/1
  Complex to Real-Imag/2 -> txQData/1

== system gm_soc_dvbs2_fpga/DVBS2/BER/Send Payload Data ==
  rst : Inport  OutDataTypeStr=boolean  PortDimensions=1  SampleTime=7.8125e-09
  nxtBit : Inport  Port=2  OutDataTypeStr=boolean  PortDimensions=1  SampleTime=7.8125e-09
  1-D Lookup Table : Subsystem
  HDL Counter : hdlsllib/Sources/HDL Counter  CountType=Count limited  CountInit=0  CountStep=1  CountMax=length([syncWord;soc_dvbs2_txPacketBits])-1  CountFromType=Initial value  CountFrom=0  CountResetPort=on  CountLoadPort=off  CountEnbPort=on  CountDirPort=off  CountHitOutputPort=off  CountDataType=Unsigned  CountWordLen=nextpow2(length([syncWord;soc_dvbs2_txPacketBits])-1)  CountFracLen=0  CountSampTime=1
  dataIn : Outport  SampleTime=7.8125e-09  InitialOutput=0  VectorParamsAs1DForOutWhenUnconnected=off
  wires:
  1-D Lookup Table/1(Out1) -> dataIn/1
  nxtBit/1 -> HDL Counter/2
  rst/1 -> HDL Counter/1
  HDL Counter/1 -> 1-D Lookup Table/1(In1)

== system gm_soc_dvbs2_fpga/DVBS2/DVBS2 TxRx/Channel ==
  txDataOut : Inport  OutDataTypeStr=fixdt(1, 18, 15)  PortDimensions=1  SampleTime=6.25e-08
      settings: SignalType=complex
  txValidOut : Inport  Port=2  OutDataTypeStr=boolean  PortDimensions=1  SampleTime=6.25e-08
  snrdB : Inport  Port=3  OutDataTypeStr=fixdt(1, 16, 9)  PortDimensions=1  SampleTime=6.25e-08
  enNoise : Inport  Port=4  OutDataTypeStr=boolean  PortDimensions=1  SampleTime=6.25e-08
  CFO : Inport  Port=5  OutDataTypeStr=fixdt(1, 21, 21)  PortDimensions=1  SampleTime=6.25e-08
  CPO : Inport  Port=6  OutDataTypeStr=fixdt(1, 21, 21)  PortDimensions=1  SampleTime=6.25e-08
  AWGN Generator : Subsystem
  Add : Sum  Inputs=+-  OutDataTypeStr=fixdt(1, 18, 15)
  Constant : Constant  Value=complex(0)  OutDataTypeStr=fixdt(1, 38, 29)  SampleTime=-1
  Data Type Conversion : DataTypeConversion  OutDataTypeStr=fixdt(1,21,0)  ConvertRealWorld=Stored Integer (SI)  SaturateOnIntegerOverflow=off  RndMeth=Floor
  Data Type Conversion1 : DataTypeConversion  OutDataTypeStr=fixdt(1,21,0)  ConvertRealWorld=Stored Integer (SI)  SaturateOnIntegerOverflow=off  RndMeth=Floor
  Delay : Delay  DelayLength=6
  NCO : dsphdlsigops2/NCO  PhaseIncrementSource=Input port  PhaseIncrement=100  PhaseOffsetSource=Input port  PhaseOffset=0  DitherSource=None  NumDitherBits=4  SamplesPerFrame=1  LUTCompress=off  ResetAction=off  Waveform=Complex exponential  PhasePort=off  SimulateUsing=Code generation  AccumulatorWL=21  PhaseQuantization=on  NumQuantizerAccumulatorBits=14  OutputDataType=Binary point scaling  OutputWL=16  OutputFL=14
  Product : Product  OutDataTypeStr=fixdt(1, 18, 15)
  Switch2 : Switch  Criteria=u2 ~= 0  OutDataTypeStr=fixdt(1, 38, 29)  SaturateOnIntegerOverflow=off  InputSameDT=off
  dataOut : Outport  SampleTime=6.25e-08
  validOut : Outport  Port=2  SampleTime=6.25e-08
  wires:
  CPO/1 -> Data Type Conversion1/1
  CFO/1 -> Data Type Conversion/1
  enNoise/1 -> Switch2/2
  AWGN Generator/1(awgn) -> Switch2/1
  snrdB/1 -> AWGN Generator/1(snrdB)
  Constant/1 -> Switch2/3
  txDataOut/1 -> Add/1
  Switch2/1 -> Add/2
  Add/1 -> Delay/1
  NCO/1 -> Product/2
  Data Type Conversion/1 -> NCO/1
  Product/1 -> dataOut/1
  Data Type Conversion1/1 -> NCO/2
  txValidOut/1 -> NCO/3
  Delay/1 -> Product/1
  NCO/2 -> validOut/1

== system gm_soc_dvbs2_fpga/DVBS2/DVBS2 TxRx/DVB-S2 HDL Receiver ==
  dataIn : Inport  OutDataTypeStr=fixdt(1, 18, 15)  PortDimensions=1  SampleTime=6.25e-08
      settings: SignalType=complex
  validIn : Inport  Port=2  OutDataTypeStr=boolean  PortDimensions=1  SampleTime=6.25e-08
  rstFCPO : Inport  Port=3  OutDataTypeStr=boolean  PortDimensions=1  SampleTime=6.25e-08
  Bus Creator : BusCreator  Inputs=11
  Bus Selector : BusSelector  OutputSignals=NormalizedCoarseFrequencyEstimate,NormalizedFineFrequencyEstimate
  Bus Selector1 : BusSelector  OutputSignals=MODCOD,FECFrame
  Bus Selector2 : BusSelector  OutputSignals=NormalizedFrequencyEstimates
  Bus Selector3 : BusSelector  OutputSignals=start,valid
  Demod Deinterleave and FECDecode : Subsystem  mask{Rsym=double(4000000), FECFrame=Short}
      mask prompts: Rsym "Symbol Rate:"; FECFrame "FEC Frame Type :"
      mask init:
      | FECFrame = double(2);
      | FECFrameConst = double(1);
      | Rsym = double(4000000);
      mask TypeOptions FECFrame: Normal | Short
      mask Display: disp(['FEC Frame Type: ' newline get_param(gcb,'FECFrame')])
  HDL Counter : hdlsllib/Sources/HDL Counter  CountType=Free running  CountInit=0  CountStep=1  CountMax=25  CountFromType=Initial value  CountFrom=0  CountResetPort=off  CountLoadPort=off  CountEnbPort=on  CountDirPort=off  CountHitOutputPort=off  CountDataType=Unsigned  CountWordLen=32  CountFracLen=0  CountSampTime=1
  Repeat1 : dspsigops/Repeat  FactorSource=Dialog parameter  N=32  Nmax=16  RateOptions=Allow multirate processing  ic=0  mode=Unused parameter value
  Stream Recovery : Subsystem  mask{Rsym=double(4000000)}
      mask prompts: Rsym "Symbol rate :"
  Synchronizer and PL Header Decoder : Subsystem  mask{Rsym=double(4000000), CFCV=off, FFCV=on, CPCV=on, FPCV=on, modcodToZero=on}
      mask prompts: Rsym "Symbol Rate :"; CFCV "Enable coarse frequency correction"; FFCV "Enable fine frequency correction"; CPCV "Enable coarse phase correction"; FPCV "Enable fine phase correction"; modcodToZero "Force MODCOD to 0 during initial synchronization"
      mask init:
      | CFCV = double(0);
      | CPCV = double(1);
      | FFCV = double(1);
      | FPCV = double(1);
      | Rsym = double(4000000);
      | config = struct('NumInputStreams', double(1), 'RolloffFactor', double(0.35), 'FilterSpanInSymbols', double(10), 'SamplesPerSymbol', double(4), 'SOFLength', double(26), 'PLSCLength', double(64), 'RRCImpulseResponse', reshape(double([0.0037515856378901708;-0.0011889692939383305;-0.0058137234310351614;-0.0051356958864536241;0.0010215774483170346;0.0066606064165017371;0.0047865298684861349;-0.0047748793834762144;-0.01272774508026017;-0.0073881081499592395;0.012808410839569809;0.032674528296556135;0.02856169072001492;-0.011037104899771699;-0.067586880212450628;-0.094323261492728655;-0.04234815425514362;0.10344298356895469;0.3039084911399606;0.47859713518808034;0.54785600668098666;0.47859713518808034;0.3039084911399606;0.10344298356895469;-0.04234815425514362;-0.094323261492728655;-0.067586880212450628;-0.011037104899771699;0.02856169072001492;0.032674528296556135;0.012808410839569809;-0.0073881081499592395;-0.01272774508026017;-0.0047748793834762144;0.0047865298684861349;0.0066606064165017371;0.0010215774483170346;-0.0051356958864536241;-0.0058137234310351614;-0.0011889692939383305;0.0037515856378901708]), [1  41]), 'refSOF', reshape(complex(double([0-0.017543859649122803i;0+0.017543859649122803i;0+0.017543859649122803i;0-0.017543859649122803i;0+0.017543859649122803i;0-0.017543859649122803i;0-0.017543859649122803i;0+0.017543859649122803i;0-0.017543859649122803i;0-0.017543859649122803i;0+0.017543859649122803i;0+0.017543859649122803i;0-0.017543859649122803i;0+0.017543859649122803i;0+0.017543859649122803i;0+0.017543859649122803i;0-0.017543859649122803i;0+0.017543859649122803i;0+0.017543859649122803i;0+0.017543859649122803i;0+0.017543859649122803i;0-0.017543859649122803i;0-0.017543859649122803i;0-0.017543859649122803i;0-0.017543859649122803i])), [1  25]), 'refPLSC', reshape(complex(double([0+0.017543859649122803i;0;0+0.017543859649122803i;0;0-0.017543859649122803i;0;0-0.017543859649122803i;0;0+0.017543859649122803i;0;0-0.017543859649122803i;0;0+0.017543859649122803i;0;0-0.017543859649122803i;0;0+0.017543859649122803i;0;0-0.017543859649122803i;0;0-0.017543859649122803i;0;0+0.017543859649122803i;0;0-0.017543859649122803i;0;0-0.017543859649122803i;0;0+0.017543859649122803i;0;0+0.017543859649122803i;0;0+0.017543859649122803i;0;0+0.017543859649122803i;0;0-0.017543859649122803i;0;0-0.017543859649122803i;0;0-0.017543859649122803i;0;0-0.017543859649122803i;0;0-0.017543859649122803i;0;0+0.017543859649122803i;0;0+0.017543859649122803i;0;0-0.017543859649122803i;0;0+0.017543859649122803i;0;0+0.017543859649122803i;0;0+0.017543859649122803i;0;0-0.017543859649122803i;0;0-0.017543859649122803i;0;0+0.017543859649122803i])), [1  63]), 'Threshold', fi(0,0,16,16,"hex","a186"), 'refSOFE', double(0.007694675284702979), 'refPLSCE', double(0.009849184364419814), 'SSKp', double(2.1560224462811557), 'SSK0', double(-1), 'SSLoopFilterPropGain', double(-0.00978978274345175), 'SSLoopFilterIntegGain', double(-0.00010442434926348536), 'PilotBlkFreq', double(16), 'SlotLength', double(90), 'nPilot', double(36), 'Pilot', complex(0.7071067811865475, 0.7071067811865475), 'PilotMinIdx', double(1440), 'PilotMaxIdx', double(1475), 'CFCLoopFilterIntegGain', double(0.0004), 'FFCAveragingLength', double(512), 'FPCLoopFilterIntegGain', double(0.00015999360025598975), 'PLSCDescramLUT', reshape(fi("numerictype",numerictype(1,2,0),"Value","[1;-1;-1;-1;1;1;1;-1;-1;1;1;-1;-1;-1;1;-1;-1;1;1;1;1;1;-1;-1;-1;-1;1;1;-1;1;1;-1;1;-1;1;-1;1;1;-1;-1;1;-1;1;1;1;1;-1;1;1;1;-1;1;-1;-1;1;-1;-1;-1;-1;-1;-1;1;-1;1]"), [64   1]), 'intColAllCodeWords1to32', reshape(uint32([1431655765;1431655765;1431677610;1431677610;1437226410;1437226410;1437248085;1437248085;1515870810;1515870810;1515890085;1515890085;1520786085;1520786085;1520805210;1520805210;1717986918;1717986918;1718000025;1718000025;1721329305;1721329305;1721342310;1721342310;1768515945;1768515945;1768527510;1768527510;1771465110;1771465110;1771476585;1771476585]), [1  32]), 'intColAllCodeWords33to64', reshape(uint32([1431655765;2863311530;1431677610;2863289685;1437226410;2857740885;1437248085;2857719210;1515870810;2779096485;1515890085;2779077210;1520786085;2774181210;1520805210;2774162085;1717986918;2576980377;1718000025;2576967270;1721329305;2573637990;1721342310;2573624985;1768515945;2526451350;1768527510;2526439785;1771465110;2523502185;1771476585;2523490710]), [1  32]), 's2xGenMatRowMask', reshape(fi("numerictype",numerictype(0,1,0),"Value","[1;0;0;1;0;0;0;0;1;0;1;0;1;1;0;0;0;0;1;0;1;1;0;1;1;1;0;1;1;1;0;1]"), [32   1]));
      | modcodToZero = double(1);
  Upsample : dspsigops/Upsample  FactorSource=Dialog parameter  N=32  Nmax=16  phase=0  RateOptions=Allow multirate processing  ic=0  mode=Unused parameter value
  Upsample1 : dspsigops/Upsample  FactorSource=Dialog parameter  N=32  Nmax=16  phase=0  RateOptions=Allow multirate processing  ic=0  mode=Unused parameter value
  Upsample2 : dspsigops/Upsample  FactorSource=Dialog parameter  N=32  Nmax=16  phase=0  RateOptions=Allow multirate processing  ic=0  mode=Unused parameter value
  bus_selector_term0 : Terminator
  syncSymb : Outport  SampleTime=2.5e-07
  syncSymbValid : Outport  Port=2  SampleTime=2.5e-07
  numSynced : Outport  Port=3  SampleTime=2.5e-07
  MODCOD : Outport  Port=4  SampleTime=2.5e-07
  fecFrame : Outport  Port=5  SampleTime=2.5e-07
  fineFreqEst : Outport  Port=6  SampleTime=2.5e-07
  bitsOut : Outport  Port=7  SampleTime=7.8125e-09  VectorParamsAs1DForOutWhenUnconnected=off
  startOut : Outport  Port=8  SampleTime=7.8125e-09  VectorParamsAs1DForOutWhenUnconnected=off
  endOut : Outport  Port=9  SampleTime=7.8125e-09  VectorParamsAs1DForOutWhenUnconnected=off
  validOut : Outport  Port=10  SampleTime=7.8125e-09  VectorParamsAs1DForOutWhenUnconnected=off
  invalidPkt : Outport  Port=11  SampleTime=7.8125e-09  VectorParamsAs1DForOutWhenUnconnected=off
  BBheaderParams : Outport  Port=12  VectorParamsAs1DForOutWhenUnconnected=off
  wires:
  Synchronizer and PL Header Decoder/5(diagBus) -> Bus Selector2/1
  Stream Recovery/10(NPD) -> Bus Creator/5  "NPD"
  rstFCPO/1 -> Synchronizer and PL Header Decoder/3(rstFCPO)
  Stream Recovery/12(MIS_ISI) -> Bus Creator/7  "MIS_ISI"
  validIn/1 -> Synchronizer and PL Header Decoder/2(validIn)
  Stream Recovery/14(DFL) -> Bus Creator/9  "DFL"
  HDL Counter/1 -> numSynced/1
  dataIn/1 -> Synchronizer and PL Header Decoder/1(dataIn)
  Bus Selector/2 -> fineFreqEst/1
  Synchronizer and PL Header Decoder/3(endOfPLSC) -> Upsample2/1, HDL Counter/1
  Synchronizer and PL Header Decoder/1(dataOut) -> Upsample/1, syncSymb/1
  Synchronizer and PL Header Decoder/4(headerInfo) -> Bus Selector1/1
  Bus Selector1/1 -> Repeat1/1, MODCOD/1
  Synchronizer and PL Header Decoder/2(validOut) -> Upsample1/1, syncSymbValid/1
  Upsample/1 -> Demod Deinterleave and FECDecode/1(dataIn)
  Stream Recovery/3(endOut) -> endOut/1
  Stream Recovery/1(bitsOut) -> bitsOut/1
  Bus Selector1/2 -> fecFrame/1
  Stream Recovery/4(validOut) -> validOut/1
  Bus Selector2/1 -> Bus Selector/1
  Upsample1/1 -> Demod Deinterleave and FECDecode/2(validIn)
  Upsample2/1 -> Demod Deinterleave and FECDecode/3(endOfPLSC)
  Demod Deinterleave and FECDecode/2(ctrl) -> Bus Selector3/1
  Repeat1/1 -> Demod Deinterleave and FECDecode/4(MODCOD)
  Bus Selector/1 -> bus_selector_term0/1
  Demod Deinterleave and FECDecode/1(bitsOut) -> Stream Recovery/1(bitsIn)
  Stream Recovery/5(invalidPkt) -> invalidPkt/1
  Bus Selector3/1 -> Stream Recovery/2(startIn)
  Bus Selector3/2 -> Stream Recovery/3(validIn)
  Stream Recovery/2(startOut) -> startOut/1
  Stream Recovery/6(TSorGS) -> Bus Creator/1  "TSorGS"
  Stream Recovery/7(SISorMIS) -> Bus Creator/2  "SISorMIS"
  Stream Recovery/8(CCMorACM) -> Bus Creator/3  "CCMorACM"
  Stream Recovery/9(ISSYI) -> Bus Creator/4  "ISSYI"
  Stream Recovery/11(RO) -> Bus Creator/6  "RO"
  Stream Recovery/13(UPL) -> Bus Creator/8  "UPL"
  Stream Recovery/15(SYNC) -> Bus Creator/10  "SYNC"
  Stream Recovery/16(SYNCD) -> Bus Creator/11  "signal11"
  Bus Creator/1 -> BBheaderParams/1

== system gm_soc_dvbs2_fpga/DVBS2/DVBS2 TxRx/Digital Automatic Gain Control ==
  dataIn : Inport  OutDataTypeStr=fixdt(1, 18, 15)  PortDimensions=1  SampleTime=6.25e-08
      settings: SignalType=complex
  validIn : Inport  Port=2  OutDataTypeStr=boolean  PortDimensions=1  SampleTime=6.25e-08
  Data Type Conversion : DataTypeConversion  OutDataTypeStr=fixdt(1, 18, 15)  SampleTime=6.25e-08  SaturateOnIntegerOverflow=off  RndMeth=Floor
  Delay{1..9} (9 alike) : Delay  DelayLength=double(2)  InitialCondition=0  SampleTime=6.25e-08
  Error Detector : Subsystem
  Loop Filter : Subsystem
  Product : Product  Inputs=**  OutDataTypeStr=fixdt(1, 55, 45)  SampleTime=6.25e-08
  dataOut : Outport  SampleTime=6.25e-08
  validOut : Outport  Port=2  SampleTime=6.25e-08
  wires:
  Delay3/1 -> Delay9/1
  validIn/1 -> Delay6/1
  dataIn/1 -> Delay7/1
  Delay4/1 -> Product/1
  Data Type Conversion/1 -> Delay2/1
  Delay6/1 -> Delay5/1
  Product/1 -> Data Type Conversion/1
  Delay5/1 -> Delay3/1
  Delay2/1 -> Delay8/1, Error Detector/1(dataIn)
  Delay7/1 -> Delay4/1
  Delay9/1 -> validOut/1
  Delay8/1 -> dataOut/1
  Error Detector/1(err) -> Loop Filter/1(err)
  Loop Filter/1(gain) -> Delay1/1
  Delay1/1 -> Product/2
